simulink library "Resident_Data"  (R2018b)
settings: Solver=ode45  StartTime=0.0  StopTime=10.0  RelTol=1e-3  EnableMultiTasking=on
settings Model: Creator=lena.frank  LastModifiedBy=drhf
settings DataIOCC: LimitDataPoints=on  SaveFormat=Array  SignalLoggingSaveFormat=ModelDataLogs
settings OptimizationCC: ExpressionDepthLimit=2147483647  LifeSpan=inf
settings DebuggingCC: UnderspecifiedInitializationDetection=Classic  MergeDetectMultiDrivingBlocksExec=none  SolverPrmCheckMsg=warning  FcnCallInpInsideContextMsg=warning  StateNameClashWarn=warning  SFUnexpectedBacktrackingDiag=warning  SFNoUnconditionalDefaultTransitionDiag=warning  SFExecutionAtInitializationDiag=none
settings HardwareCC: ProdBitPerPointer=32  ProdBitPerSizeT=32  ProdBitPerPtrDiffT=32  ProdLargestAtomicFloat=None  ProdIntDivRoundTo=Undefined  ProdEndianess=Unspecified  ProdWordSize=32  ProdHWDeviceType=32-bit Generic
settings ModelReferenceCC: PropagateSignalLabelsOutOfModel=off
settings SFSimCC: SimUseLocalCustomCode=off
settings RTWCC: RTWUseLocalCustomCode=off
settings CodeAppCC: StateflowObjectComments=on
settings GRTTargetCC: TargetLangStandard=C89/C90 (ANSI)  GeneratePreprocessorConditionals=Disable all  CombineOutputUpdateFcns=off  GRTInterface=on
settings ConfigComp: CovMetricSettings=dw  CovHtmlReporting=on  CovSaveCumulativeToWorkspaceVar=on  CovSaveSingleToWorkspaceVar=on  CovExternalEMLEnable=off

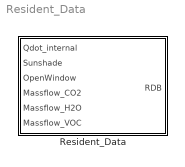
== system Resident_Data ==
  Resident_Data : Subsystem  mask(Resident Task){CalcAirComp=on}
      mask prompts: CalcAirComp "Calculate the composition of room air (H2O, CO2, VOC)"
      mask help:
      | Create the Resident Data Bus.
      | Qdot_internal : internal gains in the building in W
      | Sunshade : shading of the windows [0..1]
      | 	0 : no shading
      | 	1 : complete shading
      | OpenWindow : open the windows [0..1]
      | 	0 : closed
      | 	1 : completely opened
      | Massflow_CO2 : massflow of CO2 generated by internal sources in kg/s
      | Massflow_H2O : massflow of HO generated by internal sources in kg/s
      | Massflow_VOC : massflow of VOCs generated by internal sources in kg/s
      mask TypeOptions CalcAirComp: CalculateAirComposition/CalcAirComp
      mask Display:
      | plot(-20,-20,100,100,[30,70,70,30,30],[80,80,30,30,80],...
      |     [65,60,40,35],[30,40,40,30],...
      |     [53,53,56,56,50,44,44,47,47],...
      |     [40,45,49,60,65,60,50,45,40],...
      |     [57,50,44],[40,34,40],...
      |     [52,53],[55,55],[47,48],[55,55],...
      |     [56,53,47,44],[51,60,60,51],[52,50,48],[49,48,49])

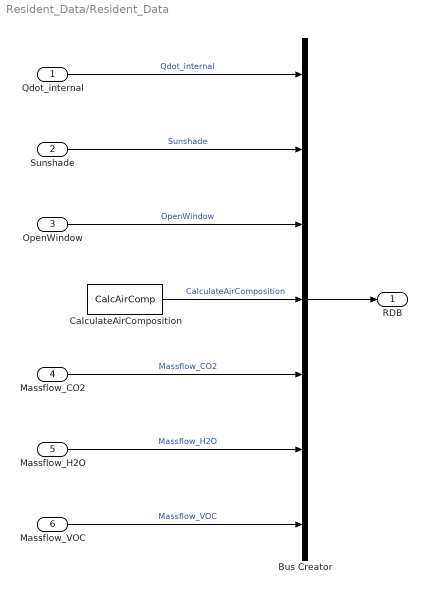
== system Resident_Data/Resident_Data ==
  Qdot_internal : Inport
  Sunshade : Inport  Port=2
  OpenWindow : Inport  Port=3
  Massflow_CO2 : Inport  Port=4
  Massflow_H2O : Inport  Port=5
  Massflow_VOC : Inport  Port=6
  Bus Creator : BusCreator  Inputs=7
  CalculateAirComposition : Constant  Value=CalcAirComp  mask{CalcAirComp=on}
      mask prompts: CalcAirComp "Calculate the composition of room air (H2O, CO2, VOC)"
  RDB : Outport
  wires:
  Sunshade/1 -> Bus Creator/2  "Sunshade"
  Bus Creator/1 -> RDB/1
  OpenWindow/1 -> Bus Creator/3  "OpenWindow"
  Qdot_internal/1 -> Bus Creator/1  "Qdot_internal"
  Massflow_CO2/1 -> Bus Creator/5  "Massflow_CO2"
  Massflow_H2O/1 -> Bus Creator/6  "Massflow_H2O"
  Massflow_VOC/1 -> Bus Creator/7  "Massflow_VOC"
  CalculateAirComposition/1 -> Bus Creator/4  "CalculateAirComposition"
